simulink model "Power_system_ZA"  (R2017a)
settings: Solver=ode45  StartTime=0.0  StopTime=tsim  RelTol=1e-3
values from neighbouring files (symbols this model uses):
  Delta_f0 = 0    [Power_system_RZA_m.m]
  Delta_P0 = 0    [Power_system_RZA_m.m]
  Delta_X0 = 0.011    [Power_system_RZA_m.m]
  denC = conv([1 0],[tauC 1])    [Power_system_RZA_m.m]
  gn = -2*Klm/Tlm/Tg    (= -1.66666666667)    [Power_system_RZA_m.m]
  Klm = 1    [Power_system_RZA_m.m]
  numC = [1.8124 -18.8558 0.1523]    [Power_system_RZA_m.m]
  psin = Klm/Tlm/Thn + Klm/Tlm/Tg    (= 0.875)    [Power_system_RZA_m.m]
  R = 0.05    [Power_system_RZA_m.m]
  Sn = 1/Thn    (= 0.25)    [Power_system_RZA_m.m]
  Tg = 0.2    [Power_system_RZA_m.m]
  Th1 = 5    [Power_system_RZA_m.m]
  Th2 = 6    [Power_system_RZA_m.m]
  Thn = 4    [Power_system_RZA_m.m]
  Tlm = 6    [Power_system_RZA_m.m]
  ttrig = 60    [Power_system_RZA_m.m]
  za0 = 0.001    [Power_system_RZA_m.m]
settings Model: Creator=Gyunghoon  LastModifiedBy=Gyunghoon
settings DataIOCC: LimitDataPoints=on  SaveFormat=Array
settings OptimizationCC: BlockReduction=off  BooleanDataType=off  LifeSpan=inf
settings DebuggingCC: SaveWithParameterizedLinksMsg=none  UnderspecifiedInitializationDetection=Classic  MergeDetectMultiDrivingBlocksExec=none  SignalResolutionControl=TryResolveAllWithWarning  SFUnexpectedBacktrackingDiag=warning  SFNoUnconditionalDefaultTransitionDiag=warning  SFExecutionAtInitializationDiag=none
settings HardwareCC: ProdBitPerPointer=32  ProdBitPerSizeT=32  ProdBitPerPtrDiffT=32  ProdLargestAtomicFloat=None  ProdIntDivRoundTo=Undefined  ProdEndianess=Unspecified  ProdWordSize=32  ProdHWDeviceType=32-bit Generic  TargetUnknown=on
settings ModelReferenceCC: PropagateSignalLabelsOutOfModel=off
settings GRTTargetCC: TargetLangStandard=C89/C90 (ANSI)  GeneratePreprocessorConditionals=Disable all
settings ConfigComp: CovMetricSettings=dw  CovHtmlReporting=on  CovSaveCumulativeToWorkspaceVar=on  CovSaveSingleToWorkspaceVar=on  CovExternalEMLEnable=off  CovSFcnEnable=off

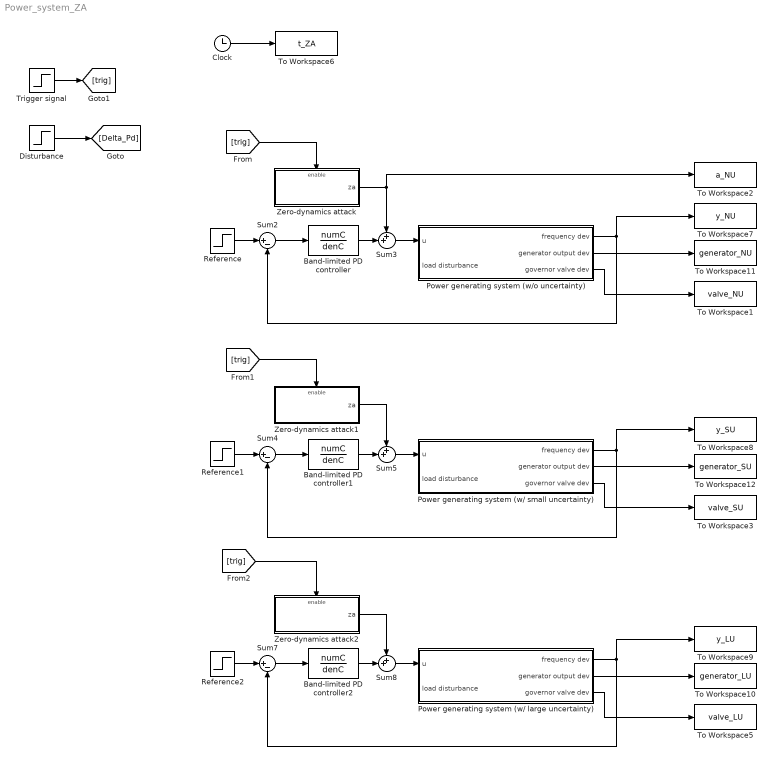
== system Power_system_ZA ==
  Band-limited PD controller : TransferFcn  Numerator=numC  Denominator=denC
  Band-limited PD controller1 : TransferFcn  Numerator=numC  Denominator=denC
  Band-limited PD controller2 : TransferFcn  Numerator=numC  Denominator=denC
  Clock : Clock
  Disturbance : Step  Time=0  After=0  SampleTime=0
  Power generating system (w/ large uncertainty) : Subsystem
  Power generating system (w/ small uncertainty) : Subsystem
  Power generating system (w/o uncertainty) : Subsystem
  Reference : Step  Time=0  After=0  SampleTime=0
  Reference1 : Step  Time=0  After=0  SampleTime=0
  Reference2 : Step  Time=0  After=0  SampleTime=0
  Sum2 : Sum  Inputs=|+-
  Sum3 : Sum  Inputs=++|
  Sum4 : Sum  Inputs=|+-
  Sum5 : Sum  Inputs=++|
  Sum7 : Sum  Inputs=|+-
  Sum8 : Sum  Inputs=++|
  To Workspace1 : ToWorkspace  VariableName=valve_NU  SampleTime=-1
  To Workspace10 : ToWorkspace  VariableName=generator_LU  SampleTime=-1
  To Workspace11 : ToWorkspace  VariableName=generator_NU  SampleTime=-1
  To Workspace12 : ToWorkspace  VariableName=generator_SU  SampleTime=-1
  To Workspace2 : ToWorkspace  VariableName=a_NU  SampleTime=-1
  To Workspace3 : ToWorkspace  VariableName=valve_SU  SampleTime=-1
  To Workspace5 : ToWorkspace  VariableName=valve_LU  SampleTime=-1
  To Workspace6 : ToWorkspace  VariableName=t_ZA  SampleTime=-1
  To Workspace7 : ToWorkspace  VariableName=y_NU  SampleTime=-1
  To Workspace8 : ToWorkspace  VariableName=y_SU  SampleTime=-1
  To Workspace9 : ToWorkspace  VariableName=y_LU  SampleTime=-1
  Trigger signal : Step  Time=ttrig  SampleTime=0
  Zero-dynamics attack : Subsystem  TreatAsAtomicUnit=on
  Zero-dynamics attack1 : Subsystem  TreatAsAtomicUnit=on
  Zero-dynamics attack2 : Subsystem  TreatAsAtomicUnit=on
  wires:
  Disturbance/1 -> [Delta_Pd]
  Power generating system (w/o uncertainty)/1(frequency dev) -> Sum2/2, To Workspace7/1
  Sum2/1 -> Band-limited PD controller/1
  Reference/1 -> Sum2/1
  Band-limited PD controller/1 -> Sum3/2
  Sum3/1 -> Power generating system (w/o uncertainty)/1(u)
  Zero-dynamics attack/1(za) -> To Workspace2/1, Sum3/1
  Power generating system (w/ small uncertainty)/1(frequency dev) -> Sum4/2, To Workspace8/1
  Sum4/1 -> Band-limited PD controller1/1
  Reference1/1 -> Sum4/1
  Band-limited PD controller1/1 -> Sum5/2
  Sum5/1 -> Power generating system (w/ small uncertainty)/1(u)
  Zero-dynamics attack1/1(za) -> Sum5/1
  Power generating system (w/ large uncertainty)/1(frequency dev) -> Sum7/2, To Workspace9/1
  Sum7/1 -> Band-limited PD controller2/1
  Reference2/1 -> Sum7/1
  Band-limited PD controller2/1 -> Sum8/2
  Sum8/1 -> Power generating system (w/ large uncertainty)/1(u)
  Zero-dynamics attack2/1(za) -> Sum8/1
  Power generating system (w/o uncertainty)/3(governor valve dev) -> To Workspace1/1
  Power generating system (w/ small uncertainty)/3(governor valve dev) -> To Workspace3/1
  Power generating system (w/ large uncertainty)/3(governor valve dev) -> To Workspace5/1
  Clock/1 -> To Workspace6/1
  Trigger signal/1 -> [trig]
  [trig] -> Zero-dynamics attack/Enable
  [trig] -> Zero-dynamics attack1/Enable
  [trig] -> Zero-dynamics attack2/Enable
  Power generating system (w/ large uncertainty)/2(generator output dev) -> To Workspace10/1
  Power generating system (w/o uncertainty)/2(generator output dev) -> To Workspace11/1
  Power generating system (w/ small uncertainty)/2(generator output dev) -> To Workspace12/1

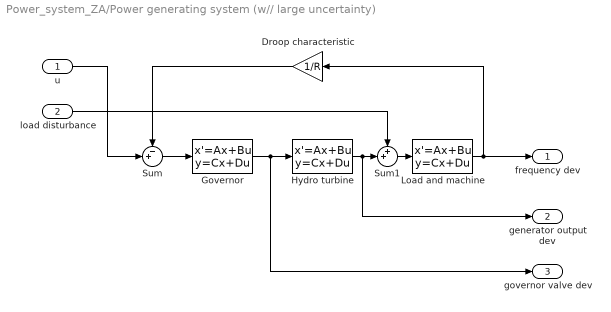
== system Power_system_ZA/Power generating system (w// large uncertainty) ==
  u : Inport
  load disturbance : Inport  Port=2
  Droop characteristic : Gain  Gain=1/R
  Governor : StateSpace  A=-1/Tg  B=1/Tg  D=0  X0=Delta_X0
  Hydro turbine : StateSpace  A=-2/Th2  B=6/Th2  D=-2  X0=Delta_P0+2*Delta_X0
  Load and machine : StateSpace  A=-1/Tlm  B=Klm/Tlm  D=0  X0=Delta_f0
  Sum : Sum  Inputs=-+|
  Sum1 : Sum  Inputs=++|
  frequency dev : Outport
  generator output dev : Outport  Port=2
  governor valve dev : Outport  Port=3
  wires:
  u/1 -> Sum/2
  Droop characteristic/1 -> Sum/1
  Load and machine/1 -> Droop characteristic/1, frequency dev/1
  Hydro turbine/1 -> generator output dev/1, Sum1/2
  Sum/1 -> Governor/1
  Governor/1 -> Hydro turbine/1, governor valve dev/1
  Sum1/1 -> Load and machine/1
  load disturbance/1 -> Sum1/1

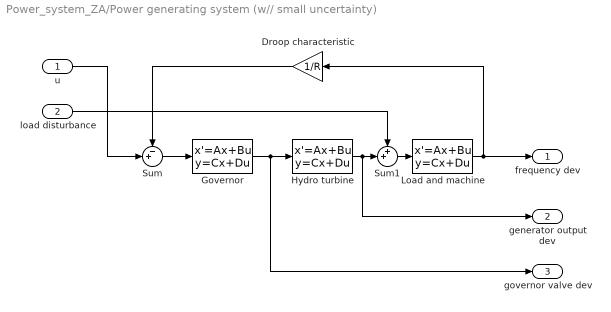
== system Power_system_ZA/Power generating system (w// small uncertainty) ==
  u : Inport
  load disturbance : Inport  Port=2
  Droop characteristic : Gain  Gain=1/R
  Governor : StateSpace  A=-1/Tg  B=1/Tg  D=0  X0=Delta_X0
  Hydro turbine : StateSpace  A=-2/Th1  B=6/Th1  D=-2  X0=Delta_P0+2*Delta_X0
  Load and machine : StateSpace  A=-1/Tlm  B=Klm/Tlm  D=0  X0=Delta_f0
  Sum : Sum  Inputs=-+|
  Sum1 : Sum  Inputs=++|
  frequency dev : Outport
  generator output dev : Outport  Port=2
  governor valve dev : Outport  Port=3
  wires:
  u/1 -> Sum/2
  Droop characteristic/1 -> Sum/1
  Load and machine/1 -> Droop characteristic/1, frequency dev/1
  Hydro turbine/1 -> generator output dev/1, Sum1/2
  Sum/1 -> Governor/1
  Governor/1 -> Hydro turbine/1, governor valve dev/1
  Sum1/1 -> Load and machine/1
  load disturbance/1 -> Sum1/1

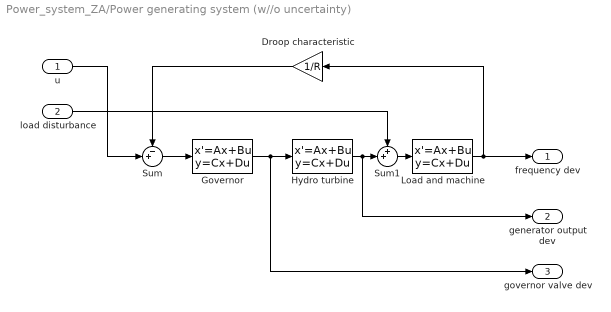
== system Power_system_ZA/Power generating system (w//o uncertainty) ==
  u : Inport
  load disturbance : Inport  Port=2
  Droop characteristic : Gain  Gain=1/R
  Governor : StateSpace  A=-1/Tg  B=1/Tg  D=0  X0=Delta_X0
  Hydro turbine : StateSpace  A=-2/Thn  B=6/Thn  D=-2  X0=Delta_P0+2*Delta_X0
  Load and machine : StateSpace  A=-1/Tlm  B=Klm/Tlm  D=0  X0=Delta_f0
  Sum : Sum  Inputs=-+|
  Sum1 : Sum  Inputs=++|
  frequency dev : Outport
  generator output dev : Outport  Port=2
  governor valve dev : Outport  Port=3
  wires:
  u/1 -> Sum/2
  Droop characteristic/1 -> Sum/1
  Load and machine/1 -> Droop characteristic/1, frequency dev/1
  Hydro turbine/1 -> generator output dev/1, Sum1/2
  Sum/1 -> Governor/1
  Governor/1 -> Hydro turbine/1, governor valve dev/1
  Sum1/1 -> Load and machine/1
  load disturbance/1 -> Sum1/1

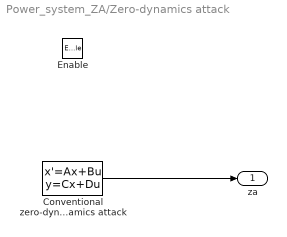
== system Power_system_ZA/Zero-dynamics attack ==
  Enable : EnablePort  PropagateVarSize=During execution
  Conventional zero-dynamics attack : StateSpace  A=Sn  B=0  C=-(1/gn)*psin  D=0  X0=za0
  za : Outport  OutputWhenDisabled=reset  InitialOutput=0
  wires:
  Conventional zero-dynamics attack/1 -> za/1

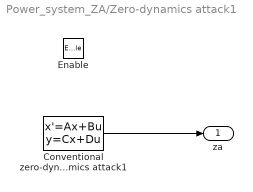
== system Power_system_ZA/Zero-dynamics attack1 ==
  Enable : EnablePort  PropagateVarSize=During execution
  Conventional zero-dynamics attack1 : StateSpace  A=Sn  B=0  C=-(1/gn)*psin  D=0  X0=za0
  za : Outport  OutputWhenDisabled=reset  InitialOutput=0
  wires:
  Conventional zero-dynamics attack1/1 -> za/1

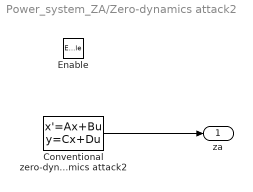
== system Power_system_ZA/Zero-dynamics attack2 ==
  Enable : EnablePort  PropagateVarSize=During execution
  Conventional zero-dynamics attack2 : StateSpace  A=Sn  B=0  C=-(1/gn)*psin  D=0  X0=za0
  za : Outport  OutputWhenDisabled=reset  InitialOutput=0
  wires:
  Conventional zero-dynamics attack2/1 -> za/1
